simulink library "ATM_lib"  (R2015a)
settings: Solver=ode45  StartTime=0.0  StopTime=10.0  RelTol=1e-3
libraries: aerolibatmos2 x1
settings Model: Creator=Andrew  LastModifiedBy=Andrew

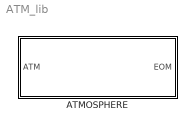
== system ATM_lib ==
  ATMOSPHERE : Subsystem

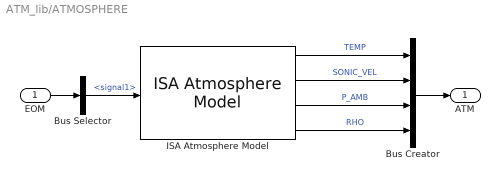
== system ATM_lib/ATMOSPHERE ==
  EOM : Inport
  Bus Creator : BusCreator
  Bus Selector : BusSelector  OutputSignals=signal1
  ISA Atmosphere Model : aerolibatmos2/ISA Atmosphere Model  custom=on  g=9.80665  gamma=1.4  R=287.0531  L=0.0065  h_trop=11000  h_strat=20000  rho0=1.225  P0=101325  T0=288.15  h0=0
  ATM : Outport
  wires:
  Bus Creator/1 -> ATM/1
  EOM/1 -> Bus Selector/1
  Bus Selector/1 -> ISA Atmosphere Model/1  "<signal1>"
  ISA Atmosphere Model/4 -> Bus Creator/4  "RHO"
  ISA Atmosphere Model/3 -> Bus Creator/3  "P_AMB"
  ISA Atmosphere Model/2 -> Bus Creator/2  "SONIC_VEL"
  ISA Atmosphere Model/1 -> Bus Creator/1  "TEMP"
